simulink model "SSRP_B"  (R2023a)
settings: Solver=FixedStepDiscrete  StartTime=0.0  StopTime=inf  RelTol=1e-3
libraries: androidcommunicationlib x3, androiduilib x2, androidaudiovideolib x1
settings Model: Creator=Lavanya  LastModifiedBy=Lavanya
settings OptimizationCC: EnhancedBackFolding=on  PassReuseOutputArgsAs=Individual arguments  ZeroExternalMemoryAtStartup=off  ZeroInternalMemoryAtStartup=off  MaxStackSize=64  OptimizeBlockOrder=speed  DifferentSizesBufferReuse=on  OptimizationCustomize=off  EfficientTunableParamExpr=on
settings DebuggingCC: ParameterTunabilityLossMsg=error
settings HardwareCC: ProdBitPerPointer=32  ProdBitPerSizeT=32  ProdBitPerPtrDiffT=32  ProdLargestAtomicInteger=Long  ProdLargestAtomicFloat=Double  ProdWordSize=32  ProdHWDeviceType=ARM Compatible->ARM Cortex  UseEmbeddedCoderFeatures=off  UseSimulinkCoderFeatures=off
settings SFSimCC: MATLABDynamicMemAlloc=off
settings RTWCC: Description=Embedded Coder  SystemTargetFile=ert.tlc  HardwareBoard=Android Device  TLCOptions="-aInlineSetEventsForThisBaseRateFcn=TLC_FALSE -aSuppressMultiTaskScheduler=TLC_FALSE  -aRateBasedStepFcn=0"  TemplateMakefile=ert_default_tmf  RTWVerbose=off  Toolchain=Android SDK/NDK Tools
settings CodeAppCC: ForceParamTrailComments=on  IgnoreCustomStorageClasses=off  OperatorAnnotations=on  SimulinkDataObjDesc=on  SFDataObjDesc=on  InsertBlockDesc=on
settings ERTTargetCC: SupportNonInlinedSFcns=on

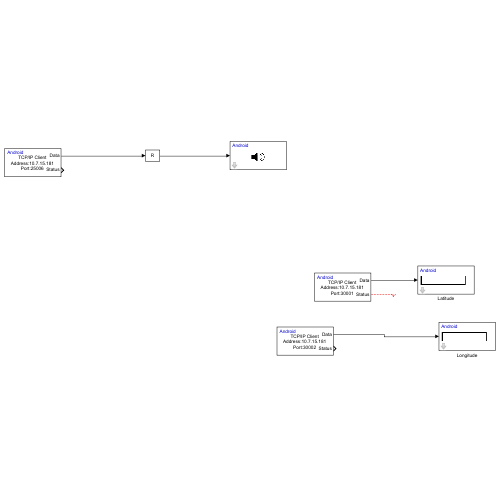
[thumbnail: Simulink's stored preview of the top-level diagram]
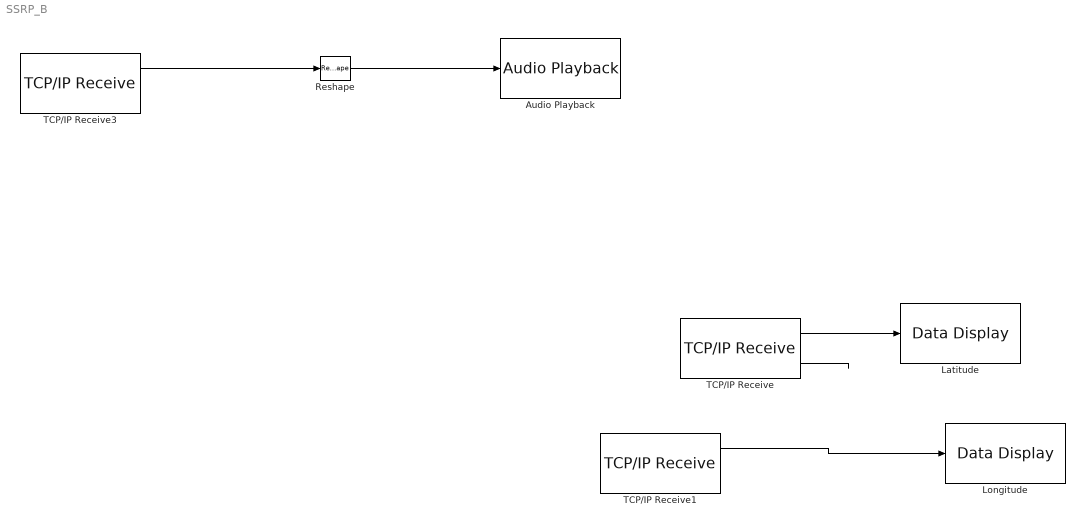
== system SSRP_B ==
  Audio Playback : androidaudiovideolib/Audio Playback  SampleFreq=44100  AudioSamplingFreq=44100  SampleTime=0.1  DeviceStr=0  QueueDuration=0  BlockPlatform=Android
  Latitude : androiduilib/Data Display  DataDisplayId=SSRP_B/Latitude  Format=Float  Precision=6  SimulateUsing=Code generation  blockPlatform=Android
  Longitude : androiduilib/Data Display  DataDisplayId=SSRP_B/Longitude  Format=Float  Precision=6  SimulateUsing=Code generation  blockPlatform=Android
  Reshape : Reshape  OutputDimensionality=Customize  OutputDimensions=[4410,2]
  TCP/IP Receive : androidcommunicationlib/TCP//IP Receive  TCPReceiveId=SSRP_B/TCP//IP_Receive  Mode_=Client  LocalServerPort_=25000  RemoteAddr_=10.7.15.181  RemoteServerPort_=30001  DataType_=double  DataSize_=1  SampleTime_=0.1  ClientPortBindingSelection_=off  ClientPortToBind_=35000  BlockingMode_=off  BlockTimeout_=0.1
  TCP/IP Receive1 : androidcommunicationlib/TCP//IP Receive  TCPReceiveId=SSRP_B/TCP//IP_Receive1  Mode_=Client  LocalServerPort_=25000  RemoteAddr_=10.7.15.181  RemoteServerPort_=30002  DataType_=double  DataSize_=1  SampleTime_=0.1  ClientPortBindingSelection_=off  ClientPortToBind_=35000  BlockingMode_=off  BlockTimeout_=0.1
  TCP/IP Receive3 : androidcommunicationlib/TCP//IP Receive  TCPReceiveId=SSRP_B/TCP//IP_Receive3  Mode_=Client  LocalServerPort_=25000  RemoteAddr_=10.7.15.181  RemoteServerPort_=25006  DataType_=int16  DataSize_=8820  SampleTime_=0.1  ClientPortBindingSelection_=off  ClientPortToBind_=35000  BlockingMode_=off  BlockTimeout_=0.1
  wires:
  TCP/IP Receive/1 -> Latitude/1
  TCP/IP Receive/2 -> ?
  TCP/IP Receive1/1 -> Longitude/1
  TCP/IP Receive3/1 -> Reshape/1
  Reshape/1 -> Audio Playback/1
